simulink model "Question2Sim"  (R2021b)
settings: Solver=VariableStepAuto  StartTime=0.0  StopTime=2  RelTol=1e-3
settings Model: Creator=Ali  LastModifiedBy=Matin

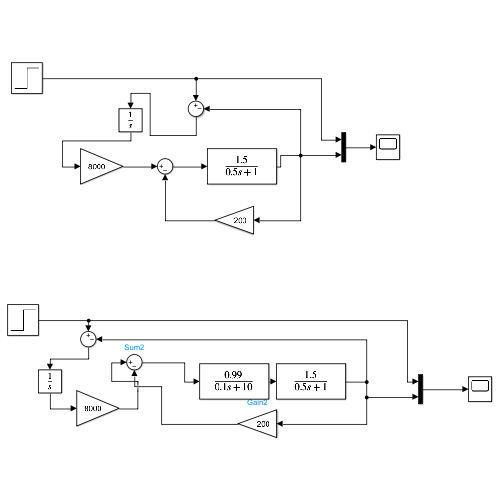
[thumbnail: Simulink's stored preview of the top-level diagram]
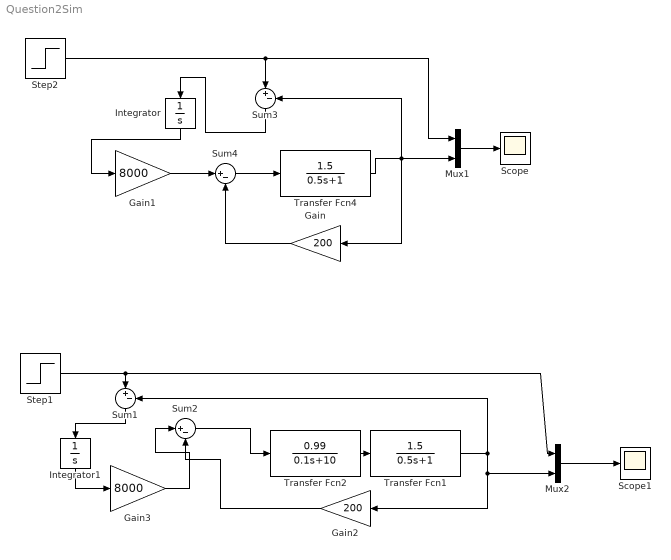
== system Question2Sim ==
  Gain : Gain  Gain=200
  Gain1 : Gain  Gain=8000
  Gain2 : Gain  Gain=200
  Gain3 : Gain  Gain=8000
  Integrator : Integrator
  Integrator1 : Integrator
  Mux1 : Mux  Inputs=2
  Mux2 : Mux  Inputs=2
  Scope : Scope
  Scope1 : Scope
  Step1 : Step  Before=0.5  After=0.6  SampleTime=0
  Step2 : Step  Before=0.5  After=0.6  SampleTime=0
  Sum{1..4} (4 alike) : Sum  Inputs=|+-
  Transfer Fcn1 : TransferFcn  Numerator=[1.5]  Denominator=[0.5 1]
  Transfer Fcn2 : TransferFcn  Numerator=[0.99]  Denominator=[0.1 10]
  Transfer Fcn4 : TransferFcn  Numerator=[1.5]  Denominator=[0.5 1]
  wires:
  Sum4/1 -> Transfer Fcn4/1
  Integrator/1 -> Gain1/1
  Mux1/1 -> Scope/1
  Gain/1 -> Sum4/2
  Gain1/1 -> Sum4/1
  Step2/1 -> Mux1/1, Sum3/1
  Transfer Fcn4/1 -> Gain/1, Sum3/2, Mux1/2
  Sum3/1 -> Integrator/1
  Transfer Fcn1/1 -> Gain2/1, Mux2/2, Sum1/2
  Gain2/1 -> Sum2/2
  Mux2/1 -> Scope1/1
  Integrator1/1 -> Gain3/1
  Gain3/1 -> Sum2/1
  Step1/1 -> Mux2/1, Sum1/1
  Sum1/1 -> Integrator1/1
  Sum2/1 -> Transfer Fcn2/1
  Transfer Fcn2/1 -> Transfer Fcn1/1
